simulink model "BEV_Laengsdynamikmodell_v2"  (R2023b)
settings: configuration reference "SharedConfig" (kept outside this file)
undefined symbols (not defined in the file): acc_cycle_flag, Analyse, battery, battery_builder_rtmsupport, config_battery, config_gearbox, config_Inverter, config_motor, config_vehicle, GB, gcbh, gearbox_map, k_FW, ModuleAssembly1, ModuleType1, motormap, motormap2
libraries: powerlib x37, nesl_utility x18, GD_Batterymodel_NSGAII_1_lib x12, BatteryProtection x9, fl_lib x7, dspstat3 x4, simulink x3, eePmsmCurrentReferenceGen x2, spsControlledCurrentSourceLib x2, spsVoltageMeasurementLib x2, batt_lib x1, BatteryBalancing x1
(part 1 of 6)
settings Model: PauseTimes=35  Creator=maximilian.tschochne  LastModifiedBy=ga58xif
settings ConfigSetRef: SourceName=SharedConfig  SourceLocation=Base Workspace

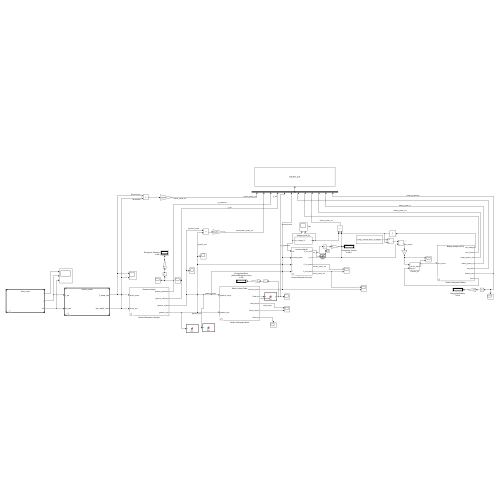
[thumbnail: Simulink's stored preview of the top-level diagram]
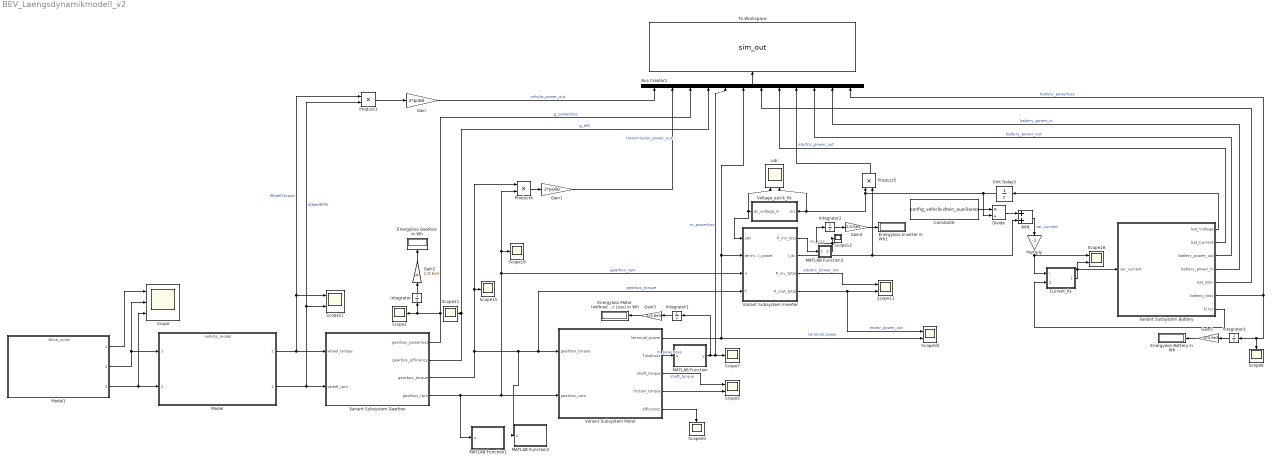
== system BEV_Laengsdynamikmodell_v2 ==
  Add : Sum
  Bus Creator1 : BusCreator  Inputs=12
  Constant6 : Constant  Value=config_vehicle.drain_auxiliaries
  Current_fix : Subsystem
  Divide : Product  Inputs=*/
  Energyloss Battery in Wh : Display
  Energyloss Gearbox in Wh : Display
  Energyloss Inverter in Wh1 : Display
  Energyloss Motor (without Mechanical Loss) in Wh : Display
  Gain : Gain  Gain=2*pi/60
  Gain1 : Gain  Gain=2*pi/60
  Gain{2..5} (4 alike) : Gain  Gain=1/3.6e3
  Integrator{,1..3} (4 alike) : Integrator
  MATLAB Function : MATLAB Function  TreatAsAtomicUnit=on
  MATLAB Function1 : MATLAB Function  TreatAsAtomicUnit=on
  MATLAB Function2 : MATLAB Function  TreatAsAtomicUnit=on
  MATLAB Function3 : MATLAB Function  TreatAsAtomicUnit=on
  Model : ModelReference  ModelNameDialog=vehicle_model.slx  SimulationMode=Normal  ModelReferenceVersion=2.0
  Model1 : ModelReference  ModelNameDialog=drive_cycle.slx  SimulationMode=Normal  ModelReferenceVersion=1.0
  Multiply : Gain  Gain=-1
  Product3 : Product
  Product4 : Product
  Product5 : Product
  Scope : Scope  NumInputPorts=3
  Scope{1,7..8,11..12,15..16,20} (8 alike) : Scope
  Scope{5,10,13,18,21} (5 alike) : Scope  NumInputPorts=2
  To Workspace : ToWorkspace  VariableName=sim_out  SaveFormat=Timeseries  SampleTime=-1
  Unit Delay3 : UnitDelay  InitialCondition=battery.SysInfo.U0_start  SampleTime=-1  HasFrameUpgradeWarning=on
  Variant Subsystem Battery : Subsystem  Variant=on
  Variant Subsystem Gearbox : Subsystem  Variant=on
  Variant Subsystem Inverter : Subsystem  Variant=on
  Variant Subsystem Motor : Subsystem  Variant=on
  Voltage_quick_fix : Subsystem
  udc : Scope  NumInputPorts=2
  wires:
  Model1/1 -> Scope/1
  Model1/2 -> Scope/2, Model/1
  Model1/3 -> Scope/3, Model/2
  Bus Creator1/1 -> To Workspace/1
  Variant Subsystem Battery/3(battery_power_out) -> Bus Creator1/10  "battery_power_out"
  Constant6/1 -> Divide/1
  Divide/1 -> Add/1
  Add/1 -> Multiply/1  "car_current"
  Gain/1 -> Bus Creator1/1  "vehicle_power_out"
  Gain1/1 -> Bus Creator1/2  "transmission_power_out"
  Model/2 -> Scope21/2, Product3/2, Variant Subsystem Gearbox/2(wheel_rpm)  "WheelRPM"
  Model/1 -> Product3/1, Scope21/1, Variant Subsystem Gearbox/1(wheel_torque)  "WheelTorque"
  Current_fix/1(car_current_batin) -> Scope18/2, Variant Subsystem Battery/1(car_current)
  Variant Subsystem Inverter/4(P_mot_total) -> Scope10/1, Scope13/2  "motor_power_out"
  Product3/1 -> Gain/1
  Product4/1 -> Gain1/1
  Variant Subsystem Inverter/3(P_inv_total) -> Scope13/1  "electric_power_out"
  Variant Subsystem Battery/4(battery_power_in) -> Bus Creator1/11  "battery_power_in"
  Variant Subsystem Gearbox/4(gearbox_rpm) -> MATLAB Function1/1(u), Variant Subsystem Motor/2(gearbox_rpm), Variant Subsystem Inverter/3(n), Scope16/1, Product4/2  "gearbox_rpm"
  Variant Subsystem Gearbox/3(gearbox_torque) -> MATLAB Function2/1(u), Variant Subsystem Inverter/4(T), Variant Subsystem Motor/1(gearbox_torque), Product4/1, Scope15/1  "gearbox_torque"
  Unit Delay3/1 -> Product5/1, udc/2, Voltage_quick_fix/1(In1), Divide/2
  Voltage_quick_fix/1(dc_voltage_in) -> Variant Subsystem Inverter/1(udc), udc/1
  Variant Subsystem Gearbox/1(gearbox_powerloss) -> Bus Creator1/3, Integrator/1, Scope1/1  "g_powerloss"
  Variant Subsystem Gearbox/2(gearbox_efficiency) -> Scope11/1, Bus Creator1/4  "g_effi"
  Variant Subsystem Inverter/1(P_inv_loss) -> MATLAB Function3/1(u)  "inv_loss"
  Multiply/1 -> Current_fix/1(i), Scope18/1
  Variant Subsystem Motor/1(terminal_power) -> Variant Subsystem Inverter/2(terminal_power), Bus Creator1/6, Scope10/2  "terminal power"
  Variant Subsystem Motor/3(shaft_torque) -> Scope5/1  "shaft_torque"
  Variant Subsystem Motor/5(efficiency) -> Scope20/1
  Integrator/1 -> Gain2/1
  Gain2/1 -> Energyloss Gearbox in Wh/1
  Gain3/1 -> Energyloss Motor (without Mechanical Loss) in Wh/1
  Integrator1/1 -> Gain3/1
  Product5/1 -> Bus Creator1/9  "electric_power_out"
  Variant Subsystem Motor/4(friction_torque) -> Scope5/2
  Variant Subsystem Battery/1(bat_Voltage) -> Unit Delay3/1
  Variant Subsystem Battery/2(bat_Current) -> Bus Creator1/8
  Variant Subsystem Battery/5(bat_SOC) -> Bus Creator1/7
  Variant Subsystem Battery/7(Error) -> Current_fix/2(flag_0V)
  Gain5/1 -> Energyloss Battery in Wh/1
  Integrator3/1 -> Gain5/1
  Variant Subsystem Battery/6(battery_loss) -> Integrator3/1, Scope8/1, Bus Creator1/12  "battery_powerloss"
  Integrator2/1 -> Gain4/1
  Gain4/1 -> Energyloss Inverter in Wh1/1
  Variant Subsystem Inverter/2(I_dc) -> Product5/2, Add/2
  MATLAB Function/1(y) -> Integrator1/1, Bus Creator1/5, Scope7/1  "m_powerloss"
  Variant Subsystem Motor/2(TotalLoss) -> MATLAB Function/1(u)  "m_powerloss"
  MATLAB Function3/1(y) -> Integrator2/1, Scope12/1

== system BEV_Laengsdynamikmodell_v2/Current_fix ==
  i : Inport
  flag_0V : Inport  Port=2
  Constant : Constant  Value=battery.SysInfo.I_max_sys
  Constant1 : Constant  Value=0
  Data Type Conversion : DataTypeConversion  OutDataTypeStr=double  SaturateOnIntegerOverflow=off  RndMeth=Floor
  MATLAB Function : MATLAB Function  TreatAsAtomicUnit=on
  MATLAB Function3 : MATLAB Function  TreatAsAtomicUnit=on
  Max : MinMax  Function=max  Inputs=2
  Min : MinMax  Inputs=2
  Scope : Scope  NumInputPorts=3
  Stop Simulation : Stop
  Switch : Switch  Criteria=u2 > Threshold  SaturateOnIntegerOverflow=off  InputSameDT=off
  Switch1 : Switch  Criteria=u2 > Threshold  SaturateOnIntegerOverflow=off  InputSameDT=off
  Unit Delay2 : UnitDelay  SampleTime=-1  HasFrameUpgradeWarning=on
  car_current_batin : Outport
  wires:
  MATLAB Function/1(y) -> Switch/2
  Min/1 -> Switch/1
  i/1 -> Switch/3, Min/2
  Constant/1 -> Min/1
  Switch1/1 -> car_current_batin/1
  Switch/1 -> Switch1/3
  Constant1/1 -> Switch1/1
  MATLAB Function3/1(y) -> Scope/1, Max/2
  Max/1 -> Scope/3, Switch1/2, Unit Delay2/1
  Unit Delay2/1 -> MATLAB Function3/1(state), Scope/2, Max/1
  flag_0V/1 -> Data Type Conversion/1
  MATLAB Function3/2(st) -> Stop Simulation/1
  Data Type Conversion/1 -> MATLAB Function3/2(u)

== system BEV_Laengsdynamikmodell_v2/Variant Subsystem Battery ==
  note: 1) Add Subsystem or Model blocks as valid variant choices.
      | 2) You cannot connect blocks at this level. At simulation, connectivity is automatically
      | determined, based on the active variant and port name matching.
  car_current : Inport
  Battery Analytic (RC3) : Subsystem  VariantControl="Battery_Mode == \"AnalyticRC3\""
  Battery Global Drive : Subsystem  VariantControl="Battery_Mode == \"Simscape\""
  Battery simplified (R0) : Subsystem  VariantControl="Battery_Mode == \"AnalyticR0\""
  bat_Voltage : Outport
  bat_Current : Outport  Port=2
  battery_power_out : Outport  Port=3
  battery_power_in : Outport  Port=4
  bat_SOC : Outport  Port=5
  battery_loss : Outport  Port=6
  Error : Outport  Port=7

== system BEV_Laengsdynamikmodell_v2/Variant Subsystem Gearbox ==
  note: 1) Add Subsystem or Model blocks as valid variant choices.
      | 2) You cannot connect blocks at this level. At simulation, connectivity is automatically
      | determined, based on the active variant and port name matching.
  wheel_torque : Inport
  wheel_rpm : Inport  Port=2
  Gearbox Analytic : Subsystem  VariantControl="GB_Mode == \"Analytic\""
  Gearbox Const : Subsystem  VariantControl="GB_Mode == \"Const\""
  Gearbox Lookup-Table : Subsystem  VariantControl="GB_Mode == \"Lookup\""
  Gearbox Simple : Subsystem  VariantControl="GB_Mode == \"Simple\""
  gearbox_powerloss : Outport
  gearbox_efficiency : Outport  Port=2
  gearbox_torque : Outport  Port=3
  gearbox_rpm : Outport  Port=4

== system BEV_Laengsdynamikmodell_v2/Variant Subsystem Inverter ==
  note: 1) Add Subsystem or Model blocks as valid variant choices.
      | 2) You cannot connect blocks at this level. At simulation, connectivity is automatically
      | determined, based on the active variant and port name matching.
  udc : Inport
  terminal_power : Inport  Port=2
  n : Inport  Port=3
  T : Inport  Port=4
  Inverter Analytic : Subsystem  VariantControl="Inverter_Mode == \"Analytic\""
  Inverter Simple : Subsystem  VariantControl="Inverter_Mode == \"Simple\""
  P_inv_loss : Outport
  I_dc : Outport  Port=2
  P_inv_total : Outport  Port=3
  P_mot_total : Outport  Port=4

== system BEV_Laengsdynamikmodell_v2/Variant Subsystem Motor ==
  note: 1) Add Subsystem or Model blocks as valid variant choices.
      | 2) You cannot connect blocks at this level. At simulation, connectivity is automatically
      | determined, based on the active variant and port name matching.
  gearbox_torque : Inport
  gearbox_rpm : Inport  Port=2
  Motor Analytic : Subsystem  VariantControl="Motor_Mode == \"Analytic\""
  Motor Const : Subsystem  VariantControl="Motor_Mode == \"Const\""
  Motor Lookup-Table : Subsystem  VariantControl="Motor_Mode == \"Lookup\""
  Motor Lookup-TableOneMotor : Subsystem  VariantControl="Motor_Mode == \"LookupOneMotor\""
  terminal_power : Outport
  TotalLoss : Outport  Port=2
  shaft_torque : Outport  Port=3
  friction_torque : Outport  Port=4
  efficiency : Outport  Port=5

== system BEV_Laengsdynamikmodell_v2/Voltage_quick_fix ==
  In1 : Inport
  Constant1 : Constant  Value=360
  MATLAB Function : MATLAB Function  TreatAsAtomicUnit=on
  Switch : Switch  Criteria=u2 > Threshold  SaturateOnIntegerOverflow=off  InputSameDT=off
  dc_voltage_in : Outport
  wires:
  Switch/1 -> dc_voltage_in/1
  MATLAB Function/1(y) -> Switch/2
  In1/1 -> Switch/3
  Constant1/1 -> Switch/1

== system BEV_Laengsdynamikmodell_v2/Variant Subsystem Battery/Battery Analytic (RC3) ==
  note: Battery model simplified by Elbadawi
  car_current : Inport
  Battery : Subsystem
  bat_Voltage : Outport
  bat_Current : Outport  Port=2
  bat_SOC : Outport  Port=3
  battery_loss : Outport  Port=4
  Error : Outport  Port=5
  battery_power_out : Outport  Port=6
  battery_power_in : Outport  Port=7
  wires:
  Battery/5(Error) -> Error/1
  Battery/4(battery_loss) -> battery_loss/1
  Battery/3(bat_SOC) -> bat_SOC/1
  Battery/2(bat_Current) -> bat_Current/1
  Battery/1(bat_Voltage) -> bat_Voltage/1
  car_current/1 -> Battery/1(car_current)
  Battery/6(battery_power_out) -> battery_power_out/1
  Battery/7(battery_power_in) -> battery_power_in/1

== system BEV_Laengsdynamikmodell_v2/Variant Subsystem Battery/Battery Global Drive ==
  car_current : Inport
  Battery : Subsystem
  bat_Voltage : Outport
  bat_Current : Outport  Port=2
  bat_SOC : Outport  Port=3
  battery_loss : Outport  Port=4
  Error : Outport  Port=5
  battery_power_out : Outport  Port=6
  battery_power_in : Outport  Port=7
  wires:
  car_current/1 -> Battery/1(car_current)
  Battery/1(bat_Voltage) -> bat_Voltage/1
  Battery/2(bat_Current) -> bat_Current/1
  Battery/3(bat_SOC) -> bat_SOC/1
  Battery/4(battery_loss) -> battery_loss/1
  Battery/5(Error) -> Error/1
  Battery/6(battery_power_out) -> battery_power_out/1
  Battery/7(battery_power_in) -> battery_power_in/1

== system BEV_Laengsdynamikmodell_v2/Variant Subsystem Battery/Battery simplified (R0) ==
  note: Battery model simplified by Elbadawi
  car_current : Inport
  Battery : Subsystem
  bat_Voltage : Outport
  bat_Current : Outport  Port=2
  bat_SOC : Outport  Port=3
  battery_loss : Outport  Port=4
  Error : Outport  Port=5
  battery_power_out : Outport  Port=6
  battery_power_in : Outport  Port=7
  wires:
  car_current/1 -> Battery/1(car_current)
  Battery/1(bat_Voltage) -> bat_Voltage/1
  Battery/2(bat_Current) -> bat_Current/1
  Battery/3(bat_SOC) -> bat_SOC/1
  Battery/4(battery_loss) -> battery_loss/1
  Battery/5(Error) -> Error/1
  Battery/6(battery_power_out) -> battery_power_out/1
  Battery/7(battery_power_in) -> battery_power_in/1

== system BEV_Laengsdynamikmodell_v2/Variant Subsystem Gearbox/Gearbox Analytic ==
  note: Wirkungsgrad:
      | Antriebsfall
  note: Sonderfall: Stillstand
  note: Sonderfall: Stillstand
  note: Wirkungsgrad:
      | Rekuperation
  wheel_rpm : Inport
  wheel_torque : Inport  Port=2
  Add : Sum
  Constant : Constant  Value=2*pi/60
  Constant1 : Constant  Value=2*pi/60
  Constant2 : Constant  Value=GB.iges
  Constant3 : Constant  Value=0
  Divide : Product  Inputs=*//
  Divide1 : Product  Inputs=*/
  Divide2 : Product  Inputs=/*
  Oil Temp : Subsystem
  Oil Temp Gao : Subsystem  Commented=on
  Product : Product
  Product1 : Product  Inputs=3
  Product2 : Product  Inputs=*/
  Saturation1 : Saturate  UpperLimit=inf  LowerLimit=0
  Scope : Scope  NumInputPorts=2
  Switch : Switch  Criteria=u2 > Threshold  SaturateOnIntegerOverflow=off  InputSameDT=off
  Switch1 : Switch  Criteria=u2 ~= 0  SaturateOnIntegerOverflow=off  InputSameDT=off
  Switch2 : Switch  Criteria=u2 ~= 0  SaturateOnIntegerOverflow=off  InputSameDT=off
  Variant Subsystem Analytic GB : Subsystem  Variant=on
  gearbox_torque : Outport
  gearbox_rpm : Outport  Port=2
  gearbox_powerloss : Outport  Port=3
  gearbox_efficiency : Outport  Port=4
  wires:
  wheel_torque/1 -> Variant Subsystem Analytic GB/1(wheel_torque), Product1/2, Product2/1, Oil Temp Gao/1(T_wheel)  "wheel_torque"
  wheel_rpm/1 -> Product/1, Variant Subsystem Analytic GB/2(wheel_rpm), Product1/3, Oil Temp Gao/2(rpm_wheel)  "wheel_rpm"
  Variant Subsystem Analytic GB/1(P_V) -> Oil Temp/1(P_V), Add/2, gearbox_powerloss/1
  Constant2/1 -> Product2/2, Product/2
  Product/1 -> Switch1/2, Divide/2, gearbox_rpm/1  "gearbox_rpm"
  Constant/1 -> Product1/1
  Product1/1 -> Divide2/1, Divide1/1, Add/1  "wheel_power"
  Add/1 -> Divide2/2, Switch/2, Divide1/2, Switch2/2, Divide/1  "gearbox_power"
  Constant1/1 -> Divide/3
  Divide/1 -> Switch1/1  "gearbox_torque_with_loss"
  Switch/1 -> Saturation1/1
  Divide2/1 -> Switch/3
  Switch1/1 -> gearbox_torque/1
  Product2/1 -> Switch1/3  "gearbox_torque_without_loss"
  Switch2/1 -> gearbox_efficiency/1
  Constant3/1 -> Switch2/3
  Divide1/1 -> Switch/1
  Oil Temp Gao/1(temp) -> Scope/1  "Temp_Gao"
  Oil Temp/1(temp) -> Scope/2, Variant Subsystem Analytic GB/3(Temp)  "Temp"
  Saturation1/1 -> Switch2/1

== system BEV_Laengsdynamikmodell_v2/Variant Subsystem Gearbox/Gearbox Const ==
  note: Rekuperation
  note: Antriebsfall
  wheel_rpm : Inport
  wheel_torque : Inport  Port=2
  Add : Sum  Inputs=-+
  Constant : Constant  Value=config_gearbox.efficiency
  Gain : Gain  Gain=2*pi/60
  Gain1 : Gain  Gain=2*pi/60
  Gearbox Ratio : Gain  Gain=config_gearbox.ratio
  Gearbox Ratio1 : Gain  Gain=1/config_gearbox.ratio
  Product : Product  Inputs=*/
  Product1 : Product  Inputs=**
  Product2 : Product
  Product3 : Product
  Switch : Switch  SaturateOnIntegerOverflow=off  InputSameDT=off
  gearbox_torque : Outport
  gearbox_rpm : Outport  Port=2
  gearbox_powerloss : Outport  Port=3
  gearbox_efficiency : Outport  Port=4
  wires:
  wheel_rpm/1 -> Product2/1, Gearbox Ratio/1
  Gearbox Ratio/1 -> gearbox_rpm/1, Product3/1  "gearbox_rpm"
  wheel_torque/1 -> Product2/2, Gearbox Ratio1/1
  Gearbox Ratio1/1 -> Product1/1, Switch/2, Product/1
  Constant/1 -> gearbox_efficiency/1, Product1/2, Product/2  "efficiency"
  Product/1 -> Switch/1
  Product1/1 -> Switch/3
  Switch/1 -> gearbox_torque/1, Product3/2  "gearbox_torque"
  Product2/1 -> Gain/1
  Add/1 -> gearbox_powerloss/1
  Product3/1 -> Gain1/1
  Gain/1 -> Add/1  "wheel_power"
  Gain1/1 -> Add/2  "gearbox_power"

== system BEV_Laengsdynamikmodell_v2/Variant Subsystem Gearbox/Gearbox Lookup-Table ==
  wheel_rpm : Inport
  wheel_torque : Inport  Port=2
  Oil Temp : Subsystem
  Oil Temp Gao : Subsystem  Commented=on
  Scope : Scope  Commented=on  NumInputPorts=2
  Variant Subsystem : Subsystem  Variant=on
  gearbox_torque : Outport
  gearbox_rpm : Outport  Port=2
  gearbox_powerloss : Outport  Port=3
  gearbox_efficiency : Outport  Port=4
  wires:
  Oil Temp Gao/1(temp) -> Scope/2
  wheel_torque/1 -> Oil Temp Gao/1(T_wheel), Variant Subsystem/1(wheel_torque)  "wheel_torque"
  wheel_rpm/1 -> Oil Temp Gao/2(rpm_wheel), Variant Subsystem/2(wheel_rpm)  "wheel_rpm"
  Variant Subsystem/4(gearbox_torque) -> gearbox_torque/1
  Variant Subsystem/1(loss_lockup) -> Oil Temp/1(P_V), gearbox_powerloss/1
  Variant Subsystem/3(gearbox_rpm) -> gearbox_rpm/1
  Variant Subsystem/2(gearbox_efficiency) -> gearbox_efficiency/1
  Oil Temp/1(temp) -> Scope/1, Variant Subsystem/3(Temp)

== system BEV_Laengsdynamikmodell_v2/Variant Subsystem Gearbox/Gearbox Simple ==
  note: Rekuperationfall
  note: Sonderfall: Ungleiche Drehmomentvorzeichen
      | Leistung nur zur Kompensation der Verluste
      | Wirkungsgrad >= 0
  note: Drehzahl und Drehmoment ungleich 0
  note: Drehmomentabhängiges
      | Verlustmoment
  note: Drehzahlabhängiges
      | Verlustmoment
  note: Wirkungsgrad nur wenn Leistung
      | übertragen wird, sonst 0
  note: Wirkungsgrad: Antriebsfall
  wheel_rpm : Inport
  wheel_torque : Inport  Port=2
  AND : Logic  Operator=OR  IconShape=distinctive  AllPortsSameDT=off  OutDataTypeStr=boolean
  Abs1 : Abs  SaturateOnIntegerOverflow=off
  Add : Sum  Inputs=-+
  Add1 : Sum  Inputs=-+++-
  Compare To Zero : simulink/Logic and Bit Operations/Compare To Zero  relop=~=  OutDataTypeStr=boolean
  Compare To Zero1 : simulink/Logic and Bit Operations/Compare To Zero  relop=~=  OutDataTypeStr=boolean
  Constant : Constant  Value=0
  Divide : Product  Inputs=/*
  Divide1 : Product  Inputs=*/
  Gain : Gain  Gain=2*pi/60
  Gain1 : Gain  Gain=config_gearbox.k_n1
  Gain2 : Gain  Gain=config_gearbox.k_M1
  Gain3 : Gain  Gain=config_gearbox.k_n2
  Gain4 : Gain  Gain=config_gearbox.k_M2
  Gain5 : Gain  Gain=2*pi/60
  Gearbox Ratio : Gain  Gain=config_gearbox.ratio
  Gearbox Ratio1 : Gain  Gain=1/config_gearbox.ratio
  Product2 : Product
  Product3 : Product
  Saturation : Saturate  UpperLimit=inf  LowerLimit=0
  Square : Math  Operator=square
  Square1 : Math  Operator=square
  Switch : Switch  Criteria=u2 > Threshold  SaturateOnIntegerOverflow=off  InputSameDT=off
  Switch1 : Switch  Criteria=u2 ~= 0  SaturateOnIntegerOverflow=off  InputSameDT=off
  gearbox_torque : Outport
  gearbox_rpm : Outport  Port=2
  gearbox_powerloss : Outport  Port=3
  gearbox_efficiency : Outport  Port=4
  wires:
  Product3/1 -> Gain5/1
  Add/1 -> gearbox_powerloss/1  "powerloss"
  Add1/1 -> Product3/2, gearbox_torque/1, Switch/2, Divide1/1, Divide/1  "gearbox_torque_with_loss"
  wheel_torque/1 -> Product2/2, Gearbox Ratio1/1
  Gearbox Ratio/1 -> Square/1, Product3/1, gearbox_rpm/1, Gain1/1  "gearbox_rpm"
  wheel_rpm/1 -> Compare To Zero/1, Gearbox Ratio/1, Product2/1
  Gearbox Ratio1/1 -> Abs1/1, Square1/1, Compare To Zero1/1, Divide1/2, Divide/2, Add1/3  "gearbox_torque_without_loss"
  Gain1/1 -> Add1/2
  Gain2/1 -> Add1/4
  Abs1/1 -> Gain2/1
  Divide/1 -> Switch/1
  Switch/1 -> Saturation/1
  Divide1/1 -> Switch/3
  Constant/1 -> Switch1/3
  Gain3/1 -> Add1/1
  Square/1 -> Gain3/1
  Switch1/1 -> gearbox_efficiency/1
  Square1/1 -> Gain4/1
  Gain4/1 -> Add1/5
  Compare To Zero1/1 -> AND/1
  Compare To Zero/1 -> AND/2
  AND/1 -> Switch1/2
  Product2/1 -> Gain/1
  Gain/1 -> Add/1  "wheel_power"
  Gain5/1 -> Add/2  "gearbox_power"
  Saturation/1 -> Switch1/1

== system BEV_Laengsdynamikmodell_v2/Variant Subsystem Inverter/Inverter Analytic ==
  udc : Inport
  n : Inport  Port=2
  T : Inport  Port=3
  terminal_power : Inport  Port=4
  Variant Subsystem : Subsystem  Variant=on
  P_inv_loss : Outport
  I_dc : Outport  Port=2
  P_inv_total : Outport  Port=3
  P_mot_total : Outport  Port=4
  wires:
  Variant Subsystem/4(P_mot_elec) -> P_mot_total/1
  Variant Subsystem/3(P_inv_total) -> P_inv_total/1
  Variant Subsystem/2(idc) -> I_dc/1
  Variant Subsystem/1(Conduction_and_Switching_loss) -> P_inv_loss/1
  T/1 -> Variant Subsystem/3(torque)
  n/1 -> Variant Subsystem/2(rpm)
  udc/1 -> Variant Subsystem/1(udc)
  terminal_power/1 -> Variant Subsystem/4(terminal_power)

== system BEV_Laengsdynamikmodell_v2/Variant Subsystem Inverter/Inverter Simple ==
  T : Inport
  n : Inport  Port=2
  udc : Inport  Port=3
  terminal_power : Inport  Port=4
  MATLAB Function : MATLAB Function  TreatAsAtomicUnit=on
  P_inv_loss : Outport
  I_dc : Outport  Port=2
  P_inv_total : Outport  Port=3
  P_mot_total : Outport  Port=4
  wires:
  T/1 -> MATLAB Function/1(T)
  n/1 -> MATLAB Function/2(n)
  udc/1 -> MATLAB Function/3(udc)
  terminal_power/1 -> MATLAB Function/4(P_Terminal)
  MATLAB Function/1(P_inv_loss) -> P_inv_loss/1
  MATLAB Function/2(I_dc) -> I_dc/1
  MATLAB Function/3(P_inv_total) -> P_inv_total/1
  MATLAB Function/4(P_mot_total) -> P_mot_total/1

== system BEV_Laengsdynamikmodell_v2/Variant Subsystem Motor/Motor Analytic ==
  note: Sonderfall:
      | keine mech. Leistung
  note: Antriebsfall
  note: Rekuperation
  note: Sonderfall: keine mech.
      | Leistung gefordert
  gearbox_torque : Inport
  gearbox_rpm : Inport  Port=2
  2-D Lookup Table : Lookup_n-D  BreakpointsForDimension1=Analyse.Betriebsdaten.M_vec(end:-1:1)  BreakpointsForDimension2=Analyse.Betriebsdaten.n_m_mesh(Analyse.Optionen.M_tics,:)  Table=Analyse.Verluste.P_vges_mesh(end:-1:1,:)  InternalRulePriority=Speed  RndMeth=Simplest
      settings: InputPortMap=u0,u1
  Add : Sum
  Add4 : Sum
  Constant1 : Constant  Value=0
  Constant2 : Constant  Value=0
  Friction & Windage : Subsystem
  Gain1 : Gain  Gain=2*pi/60
  Product : Product
  Product1 : Product  Inputs=*/
  Product2 : Product  Inputs=*/
  Saturation : Saturate  UpperLimit=inf  LowerLimit=0
  Scope1 : Scope  NumInputPorts=2
  Switch : Switch  Criteria=u2 > Threshold  SaturateOnIntegerOverflow=off  InputSameDT=off
  Switch1 : Switch  Criteria=u2 ~= 0  SaturateOnIntegerOverflow=off  InputSameDT=off
  Switch2 : Switch  Criteria=u2 ~= 0  SaturateOnIntegerOverflow=off  InputSameDT=off
  terminal_power : Outport
  TotalLoss : Outport  Port=2
  shaft_torque : Outport  Port=3
  friction_torque : Outport  Port=4
  efficiency : Outport  Port=5
  wires:
  gearbox_rpm/1 -> Friction & Windage/1(gearbox_rpm), Scope1/2, 2-D Lookup Table/2, Gain1/1  "gearbox_rpm"
  2-D Lookup Table/1 -> Add/1, TotalLoss/1  "powerloss"
  Product/1 -> Switch2/2, Product2/2, Switch1/2, Add/2, Product1/1  "power_mech"
  Add/1 -> Switch1/1, Product2/1, Switch/2, Product1/2  "power_elec"
  Product2/1 -> Switch/3
  Add4/1 -> Scope1/1, Product/1, shaft_torque/1, 2-D Lookup Table/1  "motor_torque"
  Switch2/1 -> efficiency/1
  Gain1/1 -> Product/2
  Constant2/1 -> Switch1/3
  Switch1/1 -> terminal_power/1  "Terminal Power"
  Product1/1 -> Switch/1
  gearbox_torque/1 -> Add4/1  "gearbox_torque"
  Friction & Windage/1(friction torque) -> friction_torque/1, Add4/2  "friction_torque"
  Switch/1 -> Saturation/1
  Constant1/1 -> Switch2/3
  Saturation/1 -> Switch2/1

== system BEV_Laengsdynamikmodell_v2/Variant Subsystem Motor/Motor Const ==
  note: Rekuperation
  note: Antriebsfall
  gearbox_torque : Inport
  gearbox_rpm : Inport  Port=2
  Add : Sum  Inputs=-+
  Constant : Constant  Value=config_motor.efficiency
  Friction & Windage : Subsystem
  Gain1 : Gain  Gain=2*pi/60
  Product : Product  Inputs=*/
  Product1 : Product  Inputs=**
  Product2 : Product
  Switch : Switch  SaturateOnIntegerOverflow=off  InputSameDT=off
  terminal_power : Outport
  TotalLoss : Outport  Port=2
  shaft_torque : Outport  Port=3
  friction_torque : Outport  Port=4
  efficiency : Outport  Port=5
  wires:
  Product2/1 -> Gain1/1
  Constant/1 -> efficiency/1, Product1/2, Product/2  "efficiency"
  Product/1 -> Switch/1
  Product1/1 -> Switch/3
  Add/1 -> TotalLoss/1  "powerloss"
  Switch/1 -> terminal_power/1, Add/2  "elec_power"
  gearbox_rpm/1 -> Friction & Windage/1(gearbox_rpm), Product2/2  "gearbox_rpm"
  Gain1/1 -> Add/1, Product1/1, Switch/2, Product/1  "mech_power"
  gearbox_torque/1 -> Product2/1, shaft_torque/1  "gearbox_torque"
  Friction & Windage/1(friction torque) -> friction_torque/1  "friction_torque"

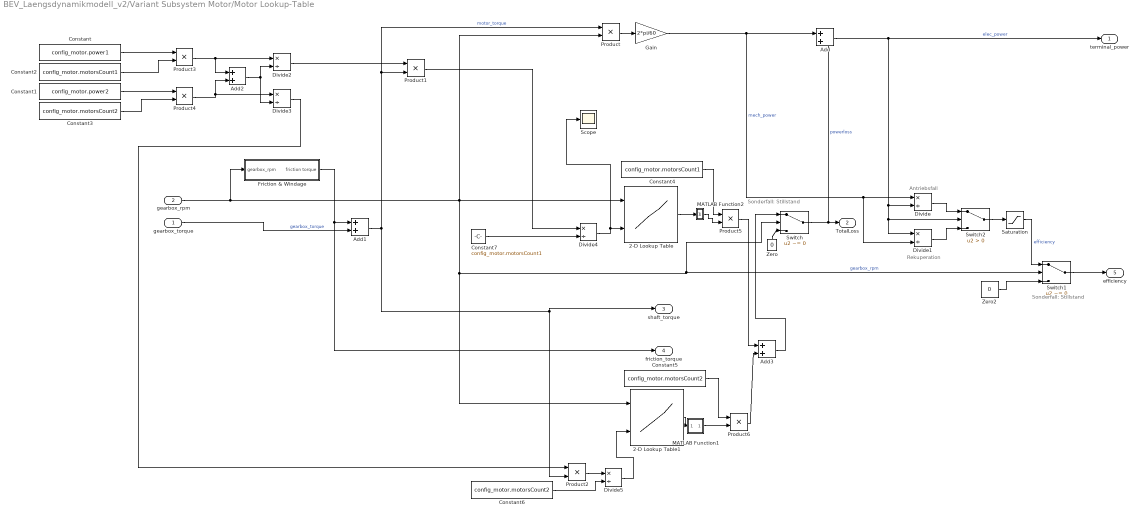
== system BEV_Laengsdynamikmodell_v2/Variant Subsystem Motor/Motor Lookup-Table ==
  note: Sonderfall: Stillstand
  note: Rekuperation
  note: Antriebsfall
  note: Sonderfall: Stillstand
  gearbox_torque : Inport
  gearbox_rpm : Inport  Port=2
  2-D Lookup Table : Lookup_n-D  BreakpointsForDimension1=motormap.nVec  BreakpointsForDimension2=motormap.MVec  Table=motormap.Loss  InternalRulePriority=Speed  RndMeth=Simplest
      settings: InputPortMap=u0,u1
  2-D Lookup Table1 : Lookup_n-D  BreakpointsForDimension1=motormap2.nVec  BreakpointsForDimension2=motormap2.MVec  Table=motormap2.Loss  InternalRulePriority=Speed  RndMeth=Simplest
      settings: InputPortMap=u0,u1
  Add{,1..3} (4 alike) : Sum
  Constant : Constant  Value=config_motor.power1
  Constant1 : Constant  Value=config_motor.power2
  Constant2 : Constant  Value=config_motor.motorsCount1
  Constant3 : Constant  Value=config_motor.motorsCount2
  Constant4 : Constant  Value=config_motor.motorsCount1
  Constant5 : Constant  Value=config_motor.motorsCount2
  Constant6 : Constant  Value=config_motor.motorsCount2
  Constant7 : Constant  Value=config_motor.motorsCount1
  Divide{,1..5} (6 alike) : Product  Inputs=*/
  Friction & Windage : Subsystem
  Gain : Gain  Gain=2*pi/60
  MATLAB Function1 : MATLAB Function  TreatAsAtomicUnit=on
  MATLAB Function2 : MATLAB Function  TreatAsAtomicUnit=on
  Product{,1..6} (7 alike) : Product
  Saturation : Saturate  UpperLimit=inf  LowerLimit=0
  Scope : Scope
  Switch : Switch  Criteria=u2 ~= 0  Threshold=1  SaturateOnIntegerOverflow=off  InputSameDT=off
  Switch1 : Switch  Criteria=u2 ~= 0  SaturateOnIntegerOverflow=off  InputSameDT=off
  Switch2 : Switch  Criteria=u2 > Threshold  SaturateOnIntegerOverflow=off  InputSameDT=off
  Zero : Constant  Value=0  OutDataTypeStr=Inherit: Inherit via back propagation
  Zero2 : Constant  Value=0  OutDataTypeStr=Inherit: Inherit via back propagation
  terminal_power : Outport
  TotalLoss : Outport  Port=2
  shaft_torque : Outport  Port=3
  friction_torque : Outport  Port=4
  efficiency : Outport  Port=5
  wires:
  Product/1 -> Gain/1
  Gain/1 -> Divide/1, Divide1/2, Add/1  "mech_power"
  Switch/1 -> TotalLoss/1, Add/2  "powerloss"
  Zero/1 -> Switch/3
  Add/1 -> Switch2/2, Divide1/1, Divide/2, terminal_power/1  "elec_power"
  Switch1/1 -> efficiency/1
  Zero2/1 -> Switch1/3
  Switch2/1 -> Saturation/1
  Divide/1 -> Switch2/1
  Divide1/1 -> Switch2/3
  Saturation/1 -> Switch1/1  "efficiency"
  gearbox_rpm/1 -> 2-D Lookup Table/1, Switch1/2, Switch/2, 2-D Lookup Table1/1, Product/2, Friction & Windage/1(gearbox_rpm)  "gearbox_rpm"
  Add1/1 -> Product2/2, shaft_torque/1, Product1/2, Product/1  "motor_torque"
  Add2/1 -> Divide3/2, Divide2/2
  Divide3/1 -> Product2/1
  Divide2/1 -> Product1/1
  2-D Lookup Table1/1 -> MATLAB Function1/1(u)
  Add3/1 -> Switch/1
  Constant/1 -> Product3/1
  2-D Lookup Table/1 -> MATLAB Function2/1(u)
  MATLAB Function2/1(y) -> Product5/2
  Constant2/1 -> Product3/2
  Constant3/1 -> Product4/2
  Constant1/1 -> Product4/1
  Product3/1 -> Divide2/1, Add2/1
  Product4/1 -> Divide3/1, Add2/2
  Product1/1 -> Divide4/1
  Product5/1 -> Add3/1
  Divide4/1 -> Scope/1, 2-D Lookup Table/2
  Product2/1 -> Divide5/1
  Divide5/1 -> 2-D Lookup Table1/2
  MATLAB Function1/1(y) -> Product6/2
  Product6/1 -> Add3/2
  Constant4/1 -> Product5/1
  Constant5/1 -> Product6/1
  Constant6/1 -> Divide5/2
  Constant7/1 -> Divide4/2
  Friction & Windage/1(friction torque) -> friction_torque/1, Add1/1
  gearbox_torque/1 -> Add1/2  "gearbox_torque"

== system BEV_Laengsdynamikmodell_v2/Variant Subsystem Motor/Motor Lookup-TableOneMotor ==
  note: Sonderfall: Stillstand
  note: Rekuperation
  note: Antriebsfall
  note: Sonderfall: Stillstand
  gearbox_torque : Inport
  gearbox_rpm : Inport  Port=2
  2-D Lookup Table : Lookup_n-D  BreakpointsForDimension1=motormap.nVec  BreakpointsForDimension2=motormap.MVec  Table=motormap.Loss  InternalRulePriority=Speed  RndMeth=Simplest
      settings: InputPortMap=u0,u1
  Add : Sum
  Add1 : Sum
  Constant1 : Constant  Value=config_motor.motorsCount1
  Constant2 : Constant  Value=config_motor.motorsCount1
  Divide : Product  Inputs=*/
  Divide1 : Product  Inputs=*/
  Divide4 : Product  Inputs=*/
  Friction & Windage : Subsystem
  Gain : Gain  Gain=2*pi/60
  MATLAB Function2 : MATLAB Function  TreatAsAtomicUnit=on
  Product : Product
  Product5 : Product
  Saturation : Saturate  UpperLimit=inf  LowerLimit=0
  Scope : Scope
  Scope1 : Scope
  Switch : Switch  Criteria=u2 ~= 0  Threshold=1  SaturateOnIntegerOverflow=off  InputSameDT=off
  Switch1 : Switch  Criteria=u2 ~= 0  SaturateOnIntegerOverflow=off  InputSameDT=off
  Switch2 : Switch  Criteria=u2 > Threshold  SaturateOnIntegerOverflow=off  InputSameDT=off
  Zero : Constant  Value=0  OutDataTypeStr=Inherit: Inherit via back propagation
  Zero2 : Constant  Value=0  OutDataTypeStr=Inherit: Inherit via back propagation
  terminal_power : Outport
  TotalLoss : Outport  Port=2
  shaft_torque : Outport  Port=3
  friction_torque : Outport  Port=4
  efficiency : Outport  Port=5
  wires:
  gearbox_torque/1 -> Add1/1  "gearbox_torque"
  Product/1 -> Gain/1
  Gain/1 -> Scope1/1, Divide/1, Divide1/2, Add/1  "mech_power"
  Switch/1 -> Add/2, Scope/1, TotalLoss/1  "powerloss"
  Zero/1 -> Switch/3
  Add/1 -> Switch2/2, Divide1/1, Divide/2, terminal_power/1  "elec_power"
  Switch1/1 -> efficiency/1
  Zero2/1 -> Switch1/3
  Switch2/1 -> Saturation/1
  Divide/1 -> Switch2/1
  Divide1/1 -> Switch2/3
  Saturation/1 -> Switch1/1  "efficiency"
  gearbox_rpm/1 -> 2-D Lookup Table/1, Switch1/2, Switch/2, Product/2, Friction & Windage/1(gearbox_rpm)  "gearbox_rpm"
  Add1/1 -> Divide4/1, shaft_torque/1, Product/1  "motor_torque"
  Friction & Windage/1(friction torque) -> friction_torque/1, Add1/2
  2-D Lookup Table/1 -> MATLAB Function2/1(u)
  MATLAB Function2/1(y) -> Product5/2
  Divide4/1 -> 2-D Lookup Table/2
  Product5/1 -> Switch/1
  Constant2/1 -> Divide4/2
  Constant1/1 -> Product5/1

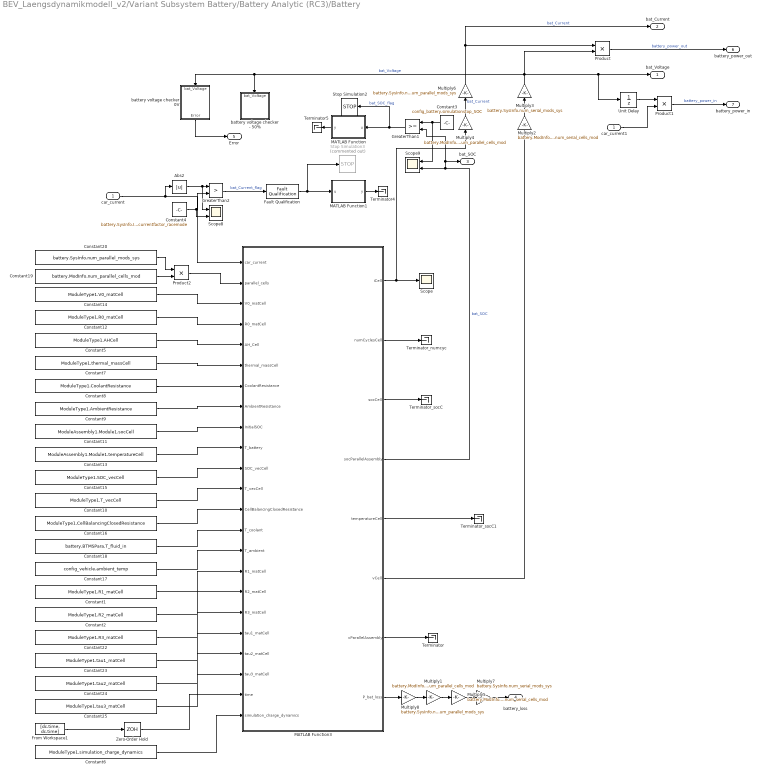
== system BEV_Laengsdynamikmodell_v2/Variant Subsystem Battery/Battery Analytic (RC3)/Battery ==
  car_current : Inport
  Abs2 : Abs  SaturateOnIntegerOverflow=off
  Constant1 : Constant  Value=ModuleType1.R1_matCell
  Constant10 : Constant  Value=ModuleType1.T_vecCell
  Constant11 : Constant  Value=ModuleAssembly1.Module1.socCell
  Constant12 : Constant  Value=ModuleType1.R0_matCell
  Constant13 : Constant  Value=ModuleAssembly1.Module1.temperatureCell
  Constant14 : Constant  Value=ModuleType1.V0_matCell
  Constant15 : Constant  Value=ModuleType1.SOC_vecCell
  Constant16 : Constant  Value=ModuleType1.CellBalancingClosedResistance
  Constant17 : Constant  Value=config_vehicle.ambient_temp
  Constant18 : Constant  Value=battery.BTMSPara.T_fluid_in
  Constant19 : Constant  Value=battery.ModInfo.num_parallel_cells_mod
  Constant2 : Constant  Value=ModuleType1.R2_matCell
  Constant20 : Constant  Value=battery.SysInfo.num_parallel_mods_sys
  Constant22 : Constant  Value=ModuleType1.R3_matCell
  Constant23 : Constant  Value=ModuleType1.tau1_matCell
  Constant24 : Constant  Value=ModuleType1.tau2_matCell
  Constant25 : Constant  Value=ModuleType1.tau3_matCell
  Constant3 : Constant  Value=config_battery.simulationstop_SOC
  Constant4 : Constant  Value=battery.SysInfo.I_max_sys * config_battery.overcurrentfactor_racemode
  Constant5 : Constant  Value=ModuleType1.AHCell
  Constant6 : Constant  Value=ModuleType1.simulation_charge_dynamics
  Constant7 : Constant  Value=ModuleType1.thermal_massCell
  Constant8 : Constant  Value=ModuleType1.CoolantResistance
  Constant9 : Constant  Value=ModuleType1.AmbientResistance
  Fault Qualification : BatteryProtection/Fault Qualification  QualTime=3  DisqualTime=6  Ts=-1
  From Workspace1 : FromWorkspace  VariableName=[dc.time, dc.time]
  GreaterThan1 : RelationalOperator  OutDataTypeStr=boolean  RndMeth=Simplest  InputSameDT=off
  GreaterThan2 : RelationalOperator  Operator=>  OutDataTypeStr=boolean  RndMeth=Simplest  InputSameDT=off
  MATLAB Function : MATLAB Function  TreatAsAtomicUnit=on
  MATLAB Function1 : MATLAB Function  TreatAsAtomicUnit=on
  MATLAB Function3 : MATLAB Function  TreatAsAtomicUnit=on
  Multiply1 : Gain  Gain=battery.ModInfo.num_parallel_cells_mod
  Multiply2 : Gain  Gain=battery.ModInfo.num_serial_cells_mod
  Multiply3 : Gain  Gain=battery.SysInfo.num_serial_mods_sys
  Multiply4 : Gain  Gain=battery.ModInfo.num_parallel_cells_mod
  Multiply5 : Gain  Gain=battery.ModInfo.num_serial_cells_mod
  Multiply6 : Gain  Gain=battery.SysInfo.num_parallel_mods_sys
  Multiply7 : Gain  Gain=battery.SysInfo.num_serial_mods_sys
  Multiply8 : Gain  Gain=battery.SysInfo.num_parallel_mods_sys
  Product : Product
  Product1 : Product
  Product2 : Product
  Scope : Scope
  Scope8 : Scope  NumInputPorts=2
  Scope9 : Scope  NumInputPorts=2
  Stop Simulation2 : Stop
  Stop Simulation3 : Stop  Commented=on
  Terminator : Terminator
  Terminator4 : Terminator
  Terminator5 : Terminator
  Terminator_numcyc : Terminator
  Terminator_socC : Terminator
  Terminator_socC1 : Terminator
  Unit Delay : UnitDelay  SampleTime=-1  HasFrameUpgradeWarning=on
  Zero-Order Hold : ZeroOrderHold  SampleTime=-1
  battery voltage checker - 50% : Subsystem
  battery voltage checker 0V : Subsystem
  car_current1 : InportShadow
  bat_Voltage : Outport
  bat_Current : Outport  Port=2
  bat_SOC : Outport  Port=3
  battery_loss : Outport  Port=4
  Error : Outport  Port=5
  battery_power_out : Outport  Port=6
  battery_power_in : Outport  Port=7
  wires:
  MATLAB Function3/5(temperatureCell) -> Terminator_socC1/1
  Product2/1 -> MATLAB Function3/2(parallel_cells)
  Constant16/1 -> MATLAB Function3/13(CellBalancingClosedResistance)
  Constant9/1 -> MATLAB Function3/8(AmbientResistance)
  Constant14/1 -> MATLAB Function3/3(V0_matCell)
  Constant13/1 -> MATLAB Function3/10(T_battery)
  Constant11/1 -> MATLAB Function3/9(InitialSOC)
  Constant15/1 -> MATLAB Function3/11(SOC_vecCell)
  Constant5/1 -> MATLAB Function3/5(AH_Cell)
  Constant12/1 -> MATLAB Function3/4(R0_matCell)
  Constant8/1 -> MATLAB Function3/7(CoolantResistance)
  Constant10/1 -> MATLAB Function3/12(T_vecCell)
  Constant7/1 -> MATLAB Function3/6(thermal_massCell)
  MATLAB Function3/2(numCyclesCell) -> Terminator_numcyc/1
  Fault Qualification/1 -> MATLAB Function1/1(u), Stop Simulation3/1
  Multiply2/1 -> Multiply3/1
  battery voltage checker 0V/1(Error) -> Error/1
  MATLAB Function3/3(socCell) -> Terminator_socC/1
  Multiply4/1 -> Multiply6/1  "bat_Current"
  MATLAB Function1/1(y) -> Terminator4/1
  MATLAB Function/1(y) -> Terminator5/1
  GreaterThan2/1 -> Fault Qualification/1  "bat_Current_flag"
  GreaterThan1/1 -> MATLAB Function/1(u), Stop Simulation2/1  "bat_SOC_flag"
  MATLAB Function3/1(iCell) -> Multiply4/1, Scope/1
  MATLAB Function3/4(socParallelAssembly) -> GreaterThan1/2, bat_SOC/1, Scope9/2  "bat_SOC"
  Constant4/1 -> GreaterThan2/2, Scope8/2
  Multiply6/1 -> bat_Current/1, Product/1  "bat_Current"
  Abs2/1 -> GreaterThan2/1, Scope8/1
  Multiply3/1 -> Product/2, battery voltage checker 0V/1(bat_Voltage), battery voltage checker - 50%/1(bat_Voltage), Unit Delay/1, bat_Voltage/1  "bat_Voltage"
  MATLAB Function3/6(vCell) -> Multiply2/1
  car_current/1 -> MATLAB Function3/1(car_current), Abs2/1
  Constant3/1 -> Scope9/1, GreaterThan1/1
  Constant2/1 -> MATLAB Function3/17(R2_matCell)
  Constant1/1 -> MATLAB Function3/16(R1_matCell)
  Constant22/1 -> MATLAB Function3/18(R3_matCell)
  Constant17/1 -> MATLAB Function3/15(T_ambient)
  Constant25/1 -> MATLAB Function3/21(tau3_matCell)
  Zero-Order Hold/1 -> MATLAB Function3/22(time)
  Constant23/1 -> MATLAB Function3/19(tau1_matCell)
  Constant18/1 -> MATLAB Function3/14(T_coolant)
  From Workspace1/1 -> Zero-Order Hold/1
  Constant24/1 -> MATLAB Function3/20(tau2_matCell)
  Unit Delay/1 -> Product1/1
  car_current1/1 -> Product1/2
  Product/1 -> battery_power_out/1  "battery_power_out"
  Product1/1 -> battery_power_in/1  "battery_power_in"
  MATLAB Function3/8(P_bat_loss) -> Multiply8/1
  MATLAB Function3/7(vParallelAssembly) -> Terminator/1
  Multiply5/1 -> Multiply7/1
  Multiply7/1 -> battery_loss/1
  Multiply1/1 -> Multiply5/1
  Constant6/1 -> MATLAB Function3/23(simulation_charge_dynamics)
  Constant19/1 -> Product2/2
  Constant20/1 -> Product2/1
  Multiply8/1 -> Multiply1/1
